simulink model "motor_cc_3"  (R2015a)
settings: Solver=ode45  StartTime=0.0  StopTime=10.0  RelTol=1e-3
values from neighbouring files (symbols this model uses):
  a = 100    [var_motor_3.m]
  Aeq = (Rou^2 - Rin^2)/2    (= 0.0002)    [var_motor_3.m]
  Bm = 0.1e-3    (= 0.0001)    [motor_lsim.m]    (also in var_motor_3.m = 0.0005)
  Bmax = 1    [var_motor_3.m]
  J = 0.2e-3    (= 0.0002)    [motor_lsim.m]    (also in var_motor_3.m = 1.5e-06)
  ks = 0.05    [var_motor_3.m]
  La = 6.6e-3    (= 0.0066)    [motor_lsim.m]    (also in var_motor_3.m = 0.0041)
  leq = 1.25e-3    (= 0.00125)    [var_motor_3.m]
  N = 100    [var_motor_3.m]
  ra = 3.15    [motor_lsim.m]    (also in var_motor_3.m = 35)
  Rp = 0.02    [var_motor_3.m]
  Tr0 = 0.175    [var_motor_3.m]
settings Model: Creator=11802972  LastModifiedBy=11802972

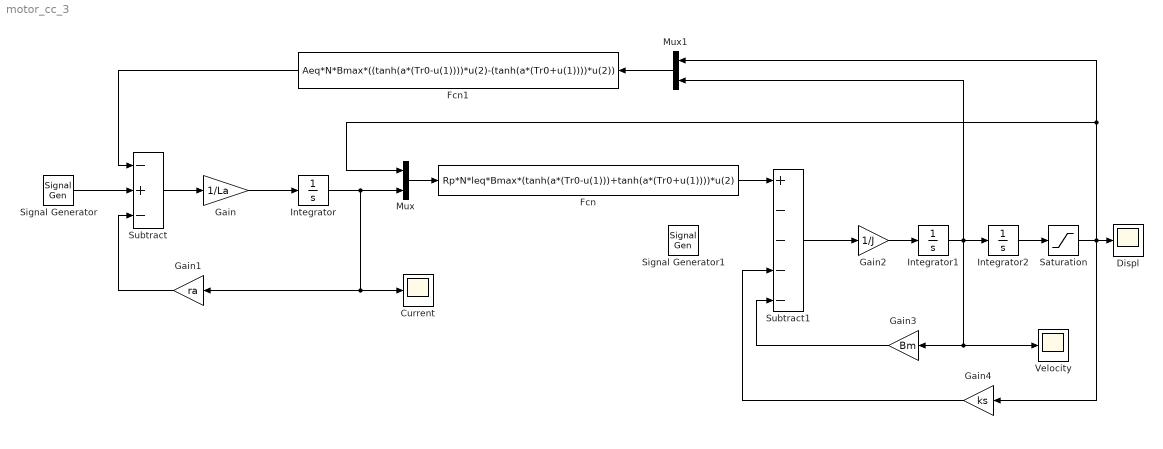
== system motor_cc_3 ==
  "Current " : Scope
  Displ : Scope
  Fcn : Fcn  Expr=Rp*N*leq*Bmax*(tanh(a*(Tr0-u(1)))+tanh(a*(Tr0+u(1))))*u(2)
  Fcn1 : Fcn  Expr=Aeq*N*Bmax*((tanh(a*(Tr0-u(1))))*u(2)-(tanh(a*(Tr0+u(1))))*u(2))
  Gain : Gain  Gain=1/La
  Gain1 : Gain  Gain=ra
  Gain2 : Gain  Gain=1/J
  Gain3 : Gain  Gain=Bm
  Gain4 : Gain  Gain=ks
  Integrator : Integrator
  Integrator1 : Integrator
  Integrator2 : Integrator
  Mux : Mux  Inputs=2
  Mux1 : Mux  Inputs=2
  Saturation : Saturate
  Signal Generator : SignalGenerator  WaveForm=square  Amplitude=-5  Frequency=10  Units=rad/sec
  Signal Generator1 : SignalGenerator  WaveForm=square  Amplitude=-5  Frequency=10  Units=rad/sec
  Subtract : Sum  Inputs=-+-
  Subtract1 : Sum  Inputs=+----
  Velocity : Scope
      settings: SaveName=ScopeData2
  wires:
  Signal Generator/1 -> Subtract/2
  Subtract/1 -> Gain/1
  Gain1/1 -> Subtract/3
  Gain/1 -> Integrator/1
  Integrator/1 -> Mux/2, "Current "/1, Gain1/1
  Mux/1 -> Fcn/1
  Fcn1/1 -> Subtract/1
  Mux1/1 -> Fcn1/1
  Gain2/1 -> Integrator1/1
  Integrator1/1 -> Mux1/2, Gain3/1, Velocity/1, Integrator2/1
  Integrator2/1 -> Saturation/1
  Saturation/1 -> Mux/1, Mux1/1, Gain4/1, Displ/1
  Fcn/1 -> Subtract1/1
  Subtract1/1 -> Gain2/1
  Gain3/1 -> Subtract1/5
  Gain4/1 -> Subtract1/4
